simulink model "SA_ACex4_ZADANIE3_1_MODEL"  (Simulink 9.1)
settings: Solver=VariableStepAuto  StartTime=0.0  StopTime=40  FixedStep=0.01  MaxStep=0.01  RelTol=1e-3  EnableMultiTasking=on
values from neighbouring files (symbols this model uses):
  omega_r = 0.25    [SA_ACex4_SKRYPT.m]
  sigma2e = 0.00    (= 0)    [SA_ACex4_SKRYPT.m]
  Ta = 0.005    [SA_ACex4_SKRYPT.m]
  Tc = 0.001    [SA_ACex4_SKRYPT.m]
  TF = 1.5*Ta    (= 0.0075)    [SA_ACex4_SKRYPT.m]
  Yr = 0.15    [SA_ACex4_SKRYPT.m]
libraries: simulink x1
settings Model: Creator=Gebruiker  LastModifiedBy=szymon
settings DataIOCC: LimitDataPoints=on  SignalLoggingSaveFormat=ModelDataLogs
settings OptimizationCC: InitFltsAndDblsToZero=on
settings DebuggingCC: SaveWithParameterizedLinksMsg=none  SignalResolutionControl=TryResolveAllWithWarning  SolverPrmCheckMsg=warning  MultiTaskDSMMsg=warning  MultiTaskCondExecSysMsg=none  FcnCallInpInsideContextMsg=warning
settings SFSimCC: SimUseLocalCustomCode=on
settings RTWCC: RTWUseLocalCustomCode=on
settings GRTTargetCC: TargetFcnLib=ansi_tfl_tmw.mat
settings ConfigComp: CovExternalEMLEnable=on

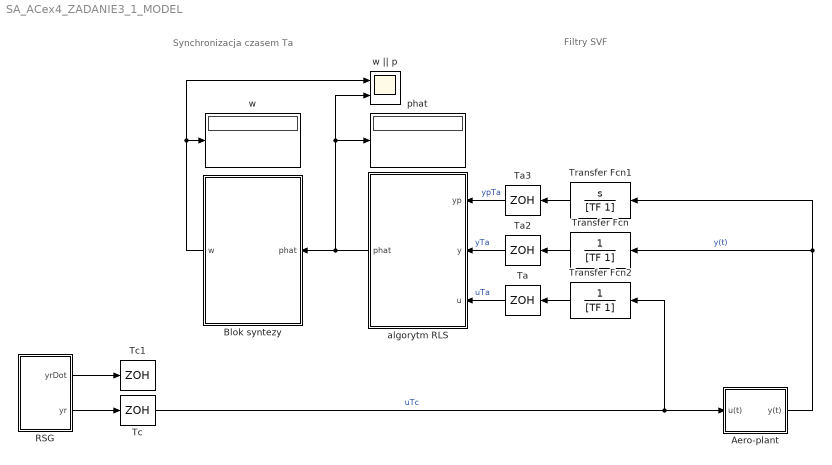
== system SA_ACex4_ZADANIE3_1_MODEL ==
  note: Synchronizacja czasem Ta
  note: Filtry SVF
  Aero-plant : Subsystem
  Blok syntezy : Subsystem
  RSG : Subsystem
  Ta : ZeroOrderHold  SampleTime=Ta
  Ta2 : ZeroOrderHold  SampleTime=Ta
  Ta3 : ZeroOrderHold  SampleTime=Ta
  Tc : ZeroOrderHold  SampleTime=Tc
  Tc1 : ZeroOrderHold  SampleTime=Tc
  Transfer Fcn : TransferFcn  Numerator=[0 1]  Denominator=[TF 1]
  Transfer Fcn1 : TransferFcn  Numerator=[1 0]  Denominator=[TF 1]
  Transfer Fcn2 : TransferFcn  Numerator=[0 1]  Denominator=[TF 1]
  algorytm RLS : Subsystem
  phat : Display
  w : Display
  w || p : Scope  NumInputPorts=2
  wires:
  Aero-plant/1(y(t)) -> Transfer Fcn1/1, Transfer Fcn/1  "y(t)"
  RSG/1(yrDot) -> Tc1/1
  RSG/2(yr) -> Tc/1
  Tc/1 -> Aero-plant/1(u(t)), Transfer Fcn2/1  "uTc"
  Transfer Fcn1/1 -> Ta3/1
  Transfer Fcn2/1 -> Ta/1
  Transfer Fcn/1 -> Ta2/1
  Ta/1 -> algorytm RLS/3(u)  "uTa"
  Ta2/1 -> algorytm RLS/2(y)  "yTa"
  Ta3/1 -> algorytm RLS/1(yp)  "ypTa"
  Blok syntezy/1(w) -> w || p/1, w/1
  algorytm RLS/1(phat) -> phat/1, w || p/2, Blok syntezy/1(phat)

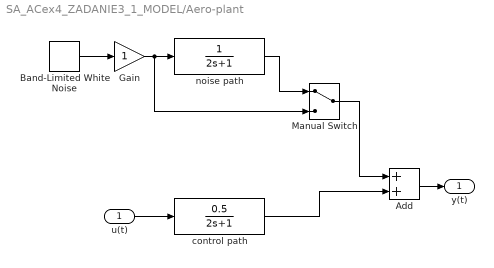
== system SA_ACex4_ZADANIE3_1_MODEL/Aero-plant ==
  u(t) : Inport
  Add : Sum
  Band-Limited White Noise : simulink/Sources/Band-Limited White Noise  Cov=[sigma2e*Tc]  Ts=Tc  seed=[23341]
  Gain : Gain
  Manual Switch : ManualSwitch
  control path : TransferFcn  Numerator=[0.5]  Denominator=[2 1]
  noise path : TransferFcn  Denominator=[2 1]
  y(t) : Outport
  wires:
  control path/1 -> Add/2
  Band-Limited White Noise/1 -> Gain/1
  Gain/1 -> Manual Switch/2, noise path/1
  Add/1 -> y(t)/1
  u(t)/1 -> control path/1
  noise path/1 -> Manual Switch/1
  Manual Switch/1 -> Add/1

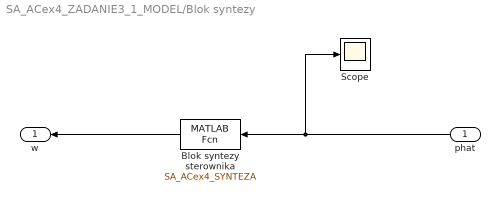
== system SA_ACex4_ZADANIE3_1_MODEL/Blok syntezy ==
  phat : Inport
  Blok syntezy sterownika : MATLABFcn  MATLABFcn=SA_ACex4_SYNTEZA
  Scope : Scope
  w : Outport
  wires:
  phat/1 -> Scope/1, Blok syntezy sterownika/1
  Blok syntezy sterownika/1 -> w/1

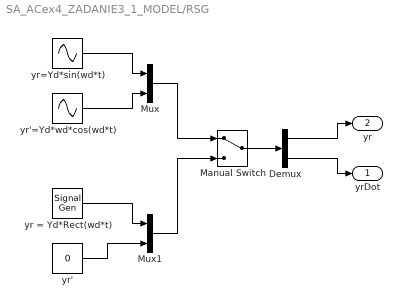
== system SA_ACex4_ZADANIE3_1_MODEL/RSG ==
  Demux : Demux  Outputs=2
  Manual Switch : ManualSwitch
  Mux : Mux  Inputs=2
  Mux1 : Mux  Inputs=2
  yr = Yd*Rect(wd*t) : SignalGenerator  WaveForm=square  Amplitude=Yr  Frequency=omega_r  Units=rad/sec
  yr' : Constant  Value=0
  yr'=Yd*wd*cos(wd*t) : Sin  Amplitude=Yr*omega_r  Frequency=omega_r  Phase=pi/2  SampleTime=0
  yr=Yd*sin(wd*t) : Sin  Amplitude=Yr  Frequency=omega_r  SampleTime=0
  yrDot : Outport
  yr : Outport  Port=2
  wires:
  yr=Yd*sin(wd*t)/1 -> Mux/1
  yr'=Yd*wd*cos(wd*t)/1 -> Mux/2
  yr = Yd*Rect(wd*t)/1 -> Mux1/1
  yr'/1 -> Mux1/2
  Mux/1 -> Manual Switch/1
  Mux1/1 -> Manual Switch/2
  Manual Switch/1 -> Demux/1
  Demux/1 -> yr/1
  Demux/2 -> yrDot/1

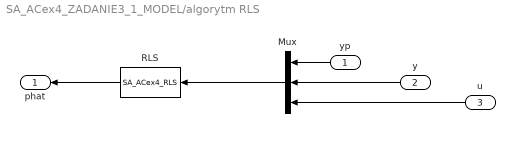
== system SA_ACex4_ZADANIE3_1_MODEL/algorytm RLS ==
  yp : Inport
  y : Inport  Port=2
  u : Inport  Port=3
  Mux : Mux  Inputs=3
  RLS : MATLABFcn  MATLABFcn=SA_ACex4_RLS  OutputDimensions=2
  phat : Outport
  wires:
  Mux/1 -> RLS/1
  RLS/1 -> phat/1
  u/1 -> Mux/3
  y/1 -> Mux/2
  yp/1 -> Mux/1
